simulink model "linear_resistor_example"  (R2025a)
settings: Solver=VariableStepAuto  StartTime=0.0  StopTime=10.0  RelTol=1e-3
libraries: nesl_utility x2
settings Model: Creator=degoede  LastModifiedBy=degoede

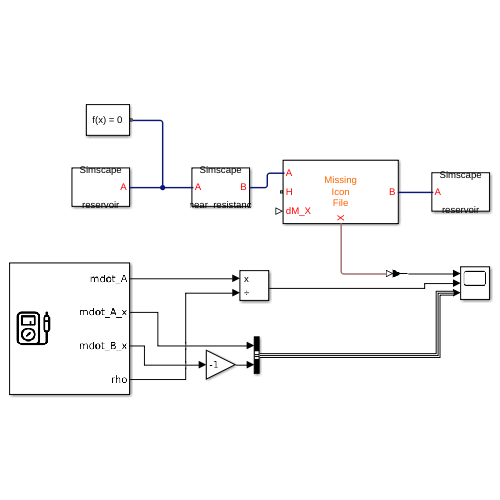
[thumbnail: Simulink's stored preview of the top-level diagram]
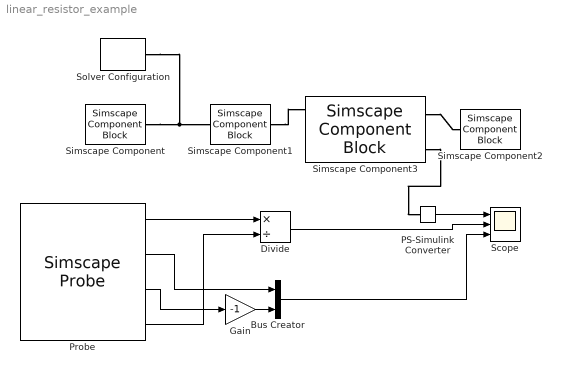
== system linear_resistor_example ==
  Bus Creator : BusCreator  Inputs=2
  Divide : Product  Inputs=*/
  Gain : Gain  Gain=-1
  PS-Simulink Converter : nesl_utility/PS-Simulink Converter  PhysicalDomain=network_engine_domain  SubClassName=ps_output  LeftPortType=input  RightPortType=output  PseudoPeriodic=off  Frequencies=[]  VectorFormat=inherit  Unit=inherit  AffineConversion=off
  Probe : SimscapeProbe  BoundBlock=2  Variables="{\"mdot_A\":{\"Probing\":\"ON\"},\"mdot_A_x\":{\"Probing\":\"ON\"},\"mdot_B_x\":{\"Probing\":\"ON\"},\"rho\":{\"Probing\":\"ON\"}}"
  Scope : Scope  NumInputPorts=3
      settings: ActiveDisplayYMinimum=0.86678590306203973  ActiveDisplayYMaximum=1.0667859030620397
  Simscape Component : SimscapeComponentBlock  SourceFile=customization.solution.elements.reservoir  ComponentPath=customization.solution.elements.reservoir  ComponentVariants="[\"customization.solution.elements.reservoir\"]"  ComponentVariantNames="[\"reservoir\"]"  ClassName=reservoir  SchemaVersion=1  pressure_spec=foundation.enum.pressure_spec.specified  reservoir_pressure=6 MPa  reservoir_temperature=293.15 K  reservoir_concentration=50 kg/m^3  area=0.01 m^2
      settings: CopyFcn=simscape.sscblock.internal.componentBlockCallback(gcbh,'COPY')  PreCopyFcn=simscape.sscblock.internal.componentBlockCallback(gcbh,'PRECOPY')  PreDeleteFcn=simscape.sscblock.internal.componentBlockCallback(gcbh,'PREDELETE')  InternalSimscapePortConfiguration="{\"Bottom\":[],\"Left\":[{\"id\":\"A\",\"label\":\"A\",\"type\":\"customization.solution.solution\"}],\"Right\":[],\"Top\":[]}"
      mask Type: Reservoir (SS)
  Simscape Component1 : SimscapeComponentBlock  SourceFile=customization.solution.elements.linear_resistance  ComponentPath=customization.solution.elements.linear_resistance  ComponentVariants="[\"customization.solution.elements.linear_resistance\"]"  ComponentVariantNames="[\"linear_resistance\"]"  ClassName=linear_resistance  SchemaVersion=1  R=6.101325e6 Pa*s/m^3  area=0.01 m^2
      settings: CopyFcn=simscape.sscblock.internal.componentBlockCallback(gcbh,'COPY')  PreCopyFcn=simscape.sscblock.internal.componentBlockCallback(gcbh,'PRECOPY')  PreDeleteFcn=simscape.sscblock.internal.componentBlockCallback(gcbh,'PREDELETE')  InternalSimscapePortConfiguration="{\"Bottom\":[],\"Left\":[{\"id\":\"A\",\"label\":\"A\",\"type\":\"customization.solution.solution\"}],\"Right\":[{\"id\":\"B\",\"label\":\"B\",\"type\":\"customization.solution.solution\"}],\"Top\":[]}"
      mask Type: Linear Resistance (SS)
  Simscape Component2 : SimscapeComponentBlock  SourceFile=customization.solution.elements.reservoir  ComponentPath=customization.solution.elements.reservoir  ComponentVariants="[\"customization.solution.elements.reservoir\"]"  ComponentVariantNames="[\"reservoir\"]"  ClassName=reservoir  SchemaVersion=1  pressure_spec=foundation.enum.pressure_spec.specified  reservoir_pressure=0.101325 MPa  reservoir_temperature=293.15 K  reservoir_concentration=0 kg/m^3  area=0.01 m^2
      settings: CopyFcn=simscape.sscblock.internal.componentBlockCallback(gcbh,'COPY')  PreCopyFcn=simscape.sscblock.internal.componentBlockCallback(gcbh,'PRECOPY')  PreDeleteFcn=simscape.sscblock.internal.componentBlockCallback(gcbh,'PREDELETE')  InternalSimscapePortConfiguration="{\"Bottom\":[],\"Left\":[{\"id\":\"A\",\"label\":\"A\",\"type\":\"customization.solution.solution\"}],\"Right\":[],\"Top\":[]}"
      mask Type: Reservoir (SS)
  Simscape Component3 : SimscapeComponentBlock  SourceFile=customization.solution.elements.constant_volume_chamber  ComponentPath=customization.solution.elements.constant_volume_chamber  ComponentVariants="[\"customization.solution.elements.constant_volume_chamber\"]"  ComponentVariantNames="[\"constant_volume_chamber\"]"  ClassName=constant_volume_chamber  SchemaVersion=1  volume=1 m^3  num_ports=foundation.enum.num_ports.two  area_A=0.01 m^2  area_B=0.01 m^2  area_C=0.01 m^2  area_D=0.01 m^2  m_measure=false  p_measure=false  t_measure=false  x_measure=true  p_I_specify=off  p_I_priority=High  p_I=0.101325 MPa  p_I_nominal_specify=off  p_I_nominal_value=1  p_I_nominal_unit=MPa  T_I_specify=off  T_I_priority=High  T_I=293.15 K  T_I_nominal_specify=off  T_I_nominal_value=1  T_I_nominal_unit=K  u_I_specify=off  u_I_priority=None  u_I=83.906 kJ/kg  u_I_nominal_specify=off  u_I_nominal_value=1  u_I_nominal_unit=kJ/kg  rho_I_specify=off  rho_I_priority=None  rho_I=998.21 kg/m^3  rho_I_nominal_specify=off  rho_I_nominal_value=1  rho_I_nominal_unit=kg/m^3  x_I_specify=off  x_I_priority=None  x_I=0 kg/m^3  x_I_nominal_specify=off  x_I_nominal_value=1  x_I_nominal_unit=kg/m^3
      settings: CopyFcn=simscape.sscblock.internal.componentBlockCallback(gcbh,'COPY')  PreCopyFcn=simscape.sscblock.internal.componentBlockCallback(gcbh,'PRECOPY')  PreDeleteFcn=simscape.sscblock.internal.componentBlockCallback(gcbh,'PREDELETE')  InternalSimscapePortConfiguration="{\"Bottom\":[{\"id\":\"X\",\"label\":\"X\",\"type\":\"output\"}],\"Left\":[{\"id\":\"A\",\"label\":\"A\",\"type\":\"customization.solution.solution\"},{\"id\":\"H\",\"label\":\"H\",\"type\":\"foundation.thermal.thermal\"},{\"id\":\"dM_X\",\"label\":\"dM_X\",\"type\":\"input\"}],\"Right\":[{\"id\":\"B\",\"label\":\"B\",\"type\":\"customization.solution.solution\"}],\"Top\":[]}"
      mask Type: Constant Volume Chamber (SS)
  Solver Configuration : nesl_utility/Solver Configuration  PhysicalDomain=network_engine_domain  SubClassName=solver  LeftPortType=input  RightPortType=generic  Tones=[]  Harmonics=[]  SimulateNoise=off  Profile=off  UseLocalSampling=off  EnableSwitchedLinearOptims=on  FrequencyDomain=off  UseCCode=off  RelTol=0.001  AbsTol=0.001  MinStep=1e-09  ToWorkspace=off  RevertToSquareIcSolve=off  NumHomotopyIterations=100  PhasorMode=off  PhasorModeNumHarmonics=1  ConsistencySolver=NEWTON_XTOL_AFTER_FTOL  IndexReductionMethod=DerivativeReplacement  DoDC=off  ResidualTolerance=1e-09  ConsistencyTolSource=GLOBAL  ConsistencyAbsTol=0.001  ConsistencyRelTol=0.001  ConsistencyTolFactor=0.001  UseLocalSolver=off  LocalSolverChoice=NE_BACKWARD_EULER_ADVANCER  ResolveIndetEquations=on  FunctionEvalNumThread=1  LocalSolverSampleTime=0.001  DoFixedCost=off  MaxNonlinIter=3  MaxModeIter=2  ComputeImpulses=off  ImpulseIterations=2  LinearAlgebra=auto  LinearAlgebraNumThread=0  EquationFormulation=NE_TIME_EF  DelaysMemoryBudget=1024  AutomaticFiltering=on  FilteringTimeConstant=0.001  PartitionStorageMethod=AS_NEEDED  PartitionMemoryBudget=1024  PartitionMethod=ROBUST  MultibodyUseLocalSolver=off  MultibodyLocalSolverChoice=ODE1  MultibodyLocalSolverSampleTime=0.001
  wires:
  Probe/1 -> Divide/1
  Probe/4 -> Divide/2
  Probe/2 -> Bus Creator/1
  Divide/1 -> Scope/2
  Bus Creator/1 -> Scope/3
  Gain/1 -> Bus Creator/2
  Probe/3 -> Gain/1
  PS-Simulink Converter/1 -> Scope/1
  connections:
  Simscape Component/LConn1 -- Solver Configuration/RConn1 -- Simscape Component1/LConn1
  Simscape Component1/RConn1 -- Simscape Component3/LConn1
  Simscape Component3/RConn1 -- Simscape Component2/LConn1
  Simscape Component3/RConn2 -- PS-Simulink Converter/LConn1
